simulink model "penduleSimple_TP2"  (R2016a)
settings: Solver=VariableStepAuto  StartTime=0.0  StopTime=10.0  RelTol=1e-3
values from neighbouring files (symbols this model uses):
  g = -9.81    [init.m]    (also in init_TP1.m; init_TP2_controle.m; init_tp3.m; matrices_init_tp4_partie3_4.m = 9.81)
  l = 10    [init.m]    (also in init_TP1.m = 1; init_TP2_controle.m; init_tp3.m = 5)
  X0 = pi/4    (= 0.785398163397)    [init.m]    (also in init_TP1.m = 0.523598775598; init_TP2_controle.m; init_tp3.m = 0.628318530718)
libraries: simulink x1
settings Model: Creator=fgaribal  LastModifiedBy=fgaribal

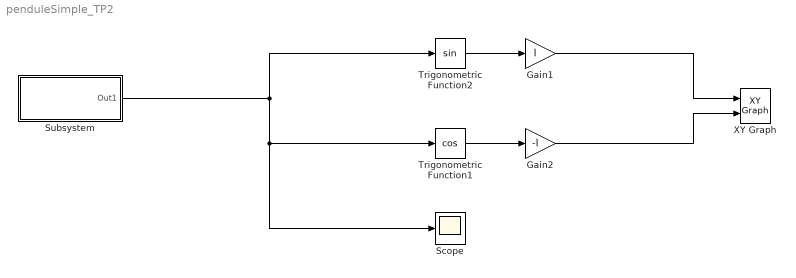
== system penduleSimple_TP2 ==
  Gain1 : Gain  Gain=l
  Gain2 : Gain  Gain=-l
  Scope : Scope
  Subsystem : Subsystem
  Trigonometric Function1 : Trigonometry  Operator=cos
  Trigonometric Function2 : Trigonometry
  XY Graph : simulink/Sinks/XY Graph  xmin=-l  xmax=l  ymin=-l  ymax=l  st=-1
  wires:
  Trigonometric Function1/1 -> Gain2/1
  Trigonometric Function2/1 -> Gain1/1
  Gain2/1 -> XY Graph/2
  Gain1/1 -> XY Graph/1
  Subsystem/1(Out1) -> Trigonometric Function1/1, Scope/1, Trigonometric Function2/1

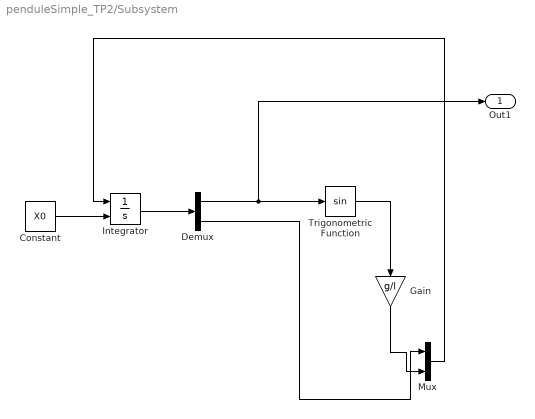
== system penduleSimple_TP2/Subsystem ==
  Constant : Constant  Value=X0
  Demux : Demux  Outputs=2
  Gain : Gain  Gain=g/l
  Integrator : Integrator  InitialConditionSource=external
  Mux : Mux  Inputs=2
  Trigonometric Function : Trigonometry
  Out1 : Outport
  wires:
  Trigonometric Function/1 -> Gain/1
  Integrator/1 -> Demux/1
  Constant/1 -> Integrator/2
  Demux/1 -> Out1/1, Trigonometric Function/1
  Demux/2 -> Mux/1
  Mux/1 -> Integrator/1
  Gain/1 -> Mux/2
